simulink model "FSK_mod_demod"  (R2021a)
settings: Solver=VariableStepAuto  StartTime=0.0  StopTime=10  RelTol=1e-3
libraries: fl_lib x93, nesl_utility x28, ee_lib x20
settings Model: Creator=Bharat Gunhalkar  LastModifiedBy=Bharat Gunhalkar

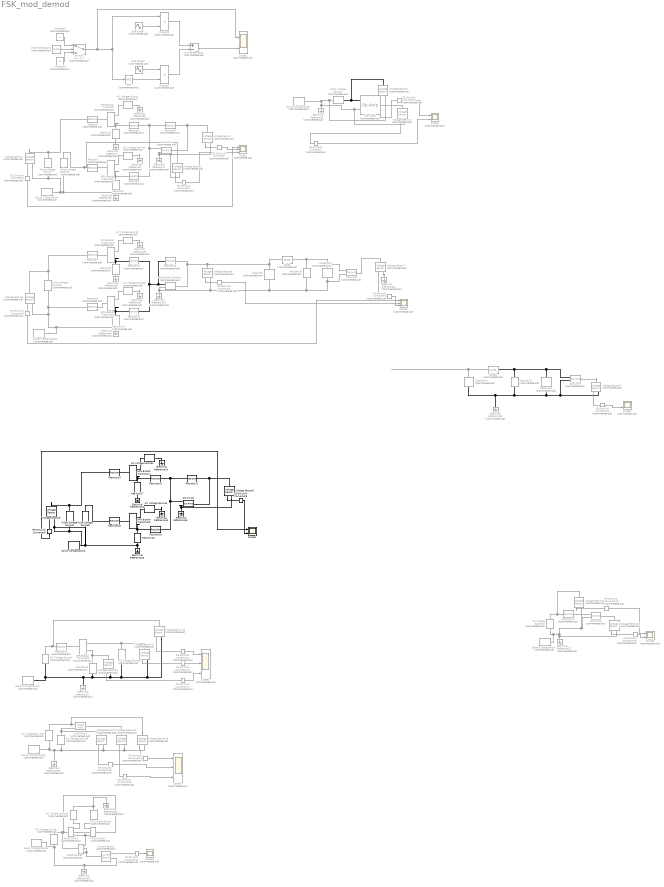
== system FSK_mod_demod ==
  AC Current Source : fl_lib/Electrical/Electrical Sources/AC Current Source  Commented=on  amp=5 A  shift=0 deg  frequency=60 Hz  omega=0 rad/s
      settings: SourceProductBaseCode=SS  InternalSimscapePortConfiguration="{\"Bottom\":[],\"Left\":[{\"id\":\"p\",\"label\":\"\",\"type\":\"foundation.electrical.electrical\"}],\"Right\":[{\"id\":\"n\",\"label\":\"\",\"type\":\"foundation.electrical.electrical\"}],\"Top\":[]}"
  AC Current Source1 : fl_lib/Electrical/Electrical Sources/AC Current Source  Commented=on  amp=2 A  shift=0 deg  frequency=60 Hz  omega=0 rad/s
      settings: SourceProductBaseCode=SS  InternalSimscapePortConfiguration="{\"Bottom\":[],\"Left\":[{\"id\":\"p\",\"label\":\"\",\"type\":\"foundation.electrical.electrical\"}],\"Right\":[{\"id\":\"n\",\"label\":\"\",\"type\":\"foundation.electrical.electrical\"}],\"Top\":[]}"
  AC Voltage Source : fl_lib/Electrical/Electrical Sources/AC Voltage Source  Commented=on  amp=.7 V  shift=90 deg  frequency=100 Hz  omega=0 rad/s
  AC Voltage Source1 : fl_lib/Electrical/Electrical Sources/AC Voltage Source  Commented=on  amp=.7 V  shift=90 deg  frequency=1000 Hz  omega=0 rad/s
  AC Voltage Source10 : fl_lib/Electrical/Electrical Sources/AC Voltage Source  Commented=on  amp=1 V  shift=0 deg  frequency=1 Hz  omega=0 rad/s
  AC Voltage Source2 : fl_lib/Electrical/Electrical Sources/AC Voltage Source  Commented=on  amp=.7 V  shift=90 deg  frequency=200 Hz  omega=0 rad/s
  AC Voltage Source3 : fl_lib/Electrical/Electrical Sources/AC Voltage Source  Commented=on  amp=.7 V  shift=90 deg  frequency=2000 Hz  omega=0 rad/s
  AC Voltage Source4 : fl_lib/Electrical/Electrical Sources/AC Voltage Source  amp=.4 V  shift=90 deg  frequency=10 Hz  omega=0 rad/s
  AC Voltage Source5 : fl_lib/Electrical/Electrical Sources/AC Voltage Source  amp=.4 V  shift=90 deg  frequency=1000 Hz  omega=0 rad/s
  AC Voltage Source6 : fl_lib/Electrical/Electrical Sources/AC Voltage Source  Commented=on  amp=4 V  shift=0 deg  frequency=.5 Hz  omega=0 rad/s
  AC Voltage Source7 : fl_lib/Electrical/Electrical Sources/AC Voltage Source  Commented=on  amp=2 V  shift=0 deg  frequency=.5 Hz  omega=0 rad/s
  AC Voltage Source8 : fl_lib/Electrical/Electrical Sources/AC Voltage Source  Commented=on  amp=2 V  shift=0 deg  frequency=.5 Hz  omega=0 rad/s
  AC Voltage Source9 : fl_lib/Electrical/Electrical Sources/AC Voltage Source  Commented=on  amp=4 V  shift=0 deg  frequency=.5 Hz  omega=0 rad/s
  CMOS AND : ee_lib/Integrated Circuits/Logic/CMOS AND  Commented=on  V_IL=2 V  V_IH=3 V  C_IN=5 pF  output_type=1  V_OL=0 V  V_OH=5 V  V_CC=5 V  V_meas=5 V  R_OUT=25 Ohm  R_OH=[25, 250] Ohm  I_OH=63 mA  R_OL=[30, 800] Ohm  I_OL=-45 mA  Delay=25 ns  Ron=5 Ohm  Vf=0.6 V  output_state=1
      settings: SourceProductBaseCode=PS  InternalSimscapePortConfiguration="{\"Bottom\":[],\"Left\":[{\"id\":\"A\",\"label\":\"\",\"type\":\"foundation.electrical.electrical\"},{\"id\":\"B\",\"label\":\"\",\"type\":\"foundation.electrical.electrical\"}],\"Right\":[{\"id\":\"J\",\"label\":\"\",\"type\":\"foundation.electrical.electrical\"}],\"Top\":[]}"
  Capacitor : fl_lib/Electrical/Electrical Elements/Capacitor  Commented=on  c=0.1e-6 F  r=1e-6 Ohm  g=0 1/Ohm  i_specify=off  i_priority=None  i=0 A  i_nominal_specify=off  i_nominal_unit=A  i_nominal_value=1  v_specify=off  v_priority=None  v=0 V  v_nominal_specify=off  v_nominal_unit=V  v_nominal_value=1  vc_specify=off  vc_priority=High  vc=0 V  vc_nominal_specify=off  vc_nominal_unit=V  vc_nominal_value=1
  Capacitor1 : fl_lib/Electrical/Electrical Elements/Capacitor  Commented=on  c=0.01e-6 F  r=1e-6 Ohm  g=0 1/Ohm  i_specify=off  i_priority=None  i=0 A  i_nominal_specify=off  i_nominal_unit=A  i_nominal_value=1  v_specify=off  v_priority=None  v=0 V  v_nominal_specify=off  v_nominal_unit=V  v_nominal_value=1  vc_specify=off  vc_priority=High  vc=0 V  vc_nominal_specify=off  vc_nominal_unit=V  vc_nominal_value=1
  Capacitor4 : fl_lib/Electrical/Electrical Elements/Capacitor  Commented=on  c=0.1 uF  r=1e-6 Ohm  g=0 1/Ohm  i_specify=off  i_priority=None  i=0 A  i_nominal_specify=off  i_nominal_unit=A  i_nominal_value=1  v_specify=off  v_priority=None  v=0 V  v_nominal_specify=off  v_nominal_unit=V  v_nominal_value=1  vc_specify=off  vc_priority=High  vc=0 V  vc_nominal_specify=off  vc_nominal_unit=V  vc_nominal_value=1
  Capacitor5 : fl_lib/Electrical/Electrical Elements/Capacitor  Commented=on  c=0.01 uF  r=1e-6 Ohm  g=0 1/Ohm  i_specify=off  i_priority=None  i=0 A  i_nominal_specify=off  i_nominal_unit=A  i_nominal_value=1  v_specify=off  v_priority=None  v=0 V  v_nominal_specify=off  v_nominal_unit=V  v_nominal_value=1  vc_specify=off  vc_priority=High  vc=0 V  vc_nominal_specify=off  vc_nominal_unit=V  vc_nominal_value=1
  Constant2 : Constant  Commented=on
  Constant3 : Constant  Commented=on  Value=0
  Current Sensor : fl_lib/Electrical/Electrical Sensors/Current Sensor  Commented=on
  DC Voltage Source : fl_lib/Electrical/Electrical Sources/DC Voltage Source  Commented=on  v0=0.5 V
  Diode : ee_lib/Semiconductors & Converters/Diode  Commented=on  ModelType=ee.enum.diode.modelType.pwl  IfMat=[.07, .12, .19, 1.75, 4.24, 7.32, 11.2; .16, .3, .72, 2.14, 5.02, 8.35, 13.12] A  TjVec=[25, 125] degC  VfVec=[.5, .7, .9, 1.3, 1.7, 2.1, 2.5] V  Vf=0.6 V  Ron=0.3 Ohm  Goff=1e-8 S  prmExp=ee.enum.diode.expParam.useTwo  I12=[.0137, .545] A  V12=[.6, .7] V  IS=1e-12 A  ec=1  I1=0.0137 A  V1=0.6 V  RS=0 Ohm  Tmeas=25 degC  N_series=1  N_parallel=1  Rz=0.3 Ohm  BV=inf V  C_param=ee.enum.diode.capParam.fixed  CJ=5 pF  CJ0=5 pF  VJ=1 V  Mgrad=0.5  Vvec=[.1, 10, 100] V  Cvec=[3.5, 1, .4] pF  FC=0.5  Q_param=ee.enum.diode.recoveryParam.off  iRM=-7.15 A  iF=4 A  didt=-750 A/us  trr_factor=3  trr=115 ns  Qrr=150 nA*s  TT=50 ns  tau=100 ns  T_param=ee.enum.diode.temperatureParam.off  IS_T2=1.25e-7 A  I1_T2=0.245 A  V1_T2=0.5 V  Tmeas2=125 degC  EG_param=ee.enum.diode.egapParam.material_si  EG=1.11 eV  XTI_param=ee.enum.diode.xtiParam.pn  XTI=3  dBVdT=0 V/K  enable_faults=simscape.enum.onoff.off  fault_action=simscape.enum.assert.action.none  fault_types=ee.enum.diode.faults.open  tau_fault=1e-3 s  IfMat_faulted=[.07, .12, .19, 1.75, 4.24, 7.32, 11.2; .16, .3, .72, 2.14, 4.02, 6.35, 9.12] A  VfVec_faulted=[.5, .7, .9, 1.3, 1.7, 2.1, 2.5] V  Ropen_faulted=1000 Ohm  Gshort_faulted=1000 1/Ohm  Vf_faulted=0.6 V  Ron_faulted=0.3 Ohm  Goff_faulted=1e-8 S  I12_faulted=[.0137, .545] A  V12_faulted=[.6, .7] V  IS_faulted=1e-12 A  ec_faulted=1  I1_faulted=0.0137 A  V1_faulted=0.6 V  RS_faulted=0 Ohm  Rz_faulted=0.3 Ohm  BV_faulted=inf V  Cscale_faulted=100  enable_temporal_fault=simscape.enum.onoff.off  t_fault=inf s  enable_behavioral_fault=simscape.enum.onoff.off  max_permissible_voltage=inf V  n_fail_on_voltage=1  max_permissible_current=inf A  t_fail_on_current=1 s  max_permissible_dVdt=inf V/s  Tdevice=25 degC  i_specify=off  i_priority=None  i=0 A  i_nominal_specify=off  i_nominal_unit=A  i_nominal_value=1  v_specify=off  v_priority=None  v=0 V  v_nominal_specify=off  v_nominal_unit=V  v_nominal_value=1  i_diode_specify=off  i_diode_priority=None  i_diode=0 A  i_diode_nominal_specify=off  i_diode_nominal_unit=A  i_diode_nominal_value=1  v_diode_specify=off  v_diode_priority=None  v_diode=0 V  v_diode_nominal_specify=off  v_diode_nominal_unit=V  v_diode_nominal_value=1  i_capacitor_specify=off  i_capacitor_priority=None  i_capacitor=0 A  i_capacitor_nominal_specify=off  i_capacitor_nominal_unit=A  i_capacitor_nominal_value=1  v_capacitor_specify=off  v_capacitor_priority=None  v_capacitor=0 V  v_capacitor_nominal_specify=off  v_capacitor_nominal_unit=V  v_capacitor_nominal_value=1  power_dissipated_specify=off  power_dissipated_priority=None  power_dissipated=0 W  power_dissipated_nominal_specify=off  power_dissipated_nominal_unit=W  power_dissipated_nominal_value=1  max_permissible_temperature=inf K  t_fail_on_temperature=1 s  thermal_network_parameterization=ee.enum.thermalNetworkTopology.junctionCase  Rth=[0, 10] K/W  Rth_Foster=[4, 6] K/W  thermal_mass_parameterization=ee.enum.thermalNetwork.timeconstant  thermal_mass=[0, 1] J/K  thermal_mass_Foster=[1.5, 3] J/K  thermal_time_constant=[0, 10] s  thermal_time_constant_Foster=[6, 18] s  thermal_mass_initial_temperatures=[25, 25] degC
  Diode2 : ee_lib/Semiconductors & Converters/Diode  Commented=on  ModelType=ee.enum.diode.modelType.pwl  IfMat=[.07, .12, .19, 1.75, 4.24, 7.32, 11.2; .16, .3, .72, 2.14, 4.02, 6.35, 9.12] A  TjVec=[25, 125] degC  VfVec=[.5, .7, .9, 1.3, 1.7, 2.1, 2.5] V  Vf=0.6 V  Ron=0.3 Ohm  Goff=1e-8 S  prmExp=ee.enum.diode.expParam.useTwo  I12=[.0137, .545] A  V12=[.6, .7] V  IS=1e-12 A  ec=1  I1=0.0137 A  V1=0.6 V  RS=0 Ohm  Tmeas=25 degC  N_series=1  N_parallel=1  Rz=0.3 Ohm  BV=inf V  C_param=ee.enum.diode.capParam.fixed  CJ=5 pF  CJ0=5 pF  VJ=1 V  Mgrad=0.5  Vvec=[.1, 10, 100] V  Cvec=[3.5, 1, .4] pF  FC=0.5  Q_param=ee.enum.diode.recoveryParam.off  iRM=-7.15 A  iF=4 A  didt=-750 A/us  trr_factor=3  trr=115 ns  Qrr=150 s*nA  TT=50 ns  tau=100 ns  T_param=ee.enum.diode.temperatureParam.off  IS_T2=1.25e-7 A  I1_T2=0.245 A  V1_T2=0.5 V  Tmeas2=125 degC  EG_param=ee.enum.diode.egapParam.material_si  EG=1.11 eV  XTI_param=ee.enum.diode.xtiParam.pn  XTI=3  dBVdT=0 V/K  enable_faults=ee.enum.faults.faultEnable.no  fault_action=ee.enum.faults.faultAction.none  fault_types=ee.enum.diode.faults.open  tau_fault=1e-3 s  IfMat_faulted=[.07, .12, .19, 1.75, 4.24, 7.32, 11.2; .16, .3, .72, 2.14, 4.02, 6.35, 9.12] A  VfVec_faulted=[.5, .7, .9, 1.3, 1.7, 2.1, 2.5] V  Ropen_faulted=1000 Ohm  Gshort_faulted=1000 1/Ohm  Vf_faulted=0.6 V  Ron_faulted=0.3 Ohm  Goff_faulted=1e-8 S  I12_faulted=[.0137, .545] A  V12_faulted=[.6, .7] V  IS_faulted=1e-12 A  ec_faulted=1  I1_faulted=0.0137 A  V1_faulted=0.6 V  RS_faulted=0 Ohm  Rz_faulted=0.3 Ohm  BV_faulted=inf V  Cscale_faulted=100  enable_temporal_fault=ee.enum.faults.faultEnable.no  t_fault=inf s  enable_behavioral_fault=ee.enum.faults.faultEnable.no  max_permissible_voltage=inf V  n_fail_on_voltage=1  max_permissible_current=inf A  t_fail_on_current=1 s  max_permissible_dVdt=inf V/s  Tdevice=25 degC  i_specify=off  i_priority=None  i=0 A  i_nominal_specify=off  i_nominal_unit=A  i_nominal_value=1  v_specify=off  v_priority=None  v=0 V  v_nominal_specify=off  v_nominal_unit=V  v_nominal_value=1  i_diode_specify=off  i_diode_priority=None  i_diode=0 A  i_diode_nominal_specify=off  i_diode_nominal_unit=A  i_diode_nominal_value=1  v_diode_specify=off  v_diode_priority=None  v_diode=0 V  v_diode_nominal_specify=off  v_diode_nominal_unit=V  v_diode_nominal_value=1  i_capacitor_specify=off  i_capacitor_priority=None  i_capacitor=0 A  i_capacitor_nominal_specify=off  i_capacitor_nominal_unit=A  i_capacitor_nominal_value=1  v_capacitor_specify=off  v_capacitor_priority=None  v_capacitor=0 V  v_capacitor_nominal_specify=off  v_capacitor_nominal_unit=V  v_capacitor_nominal_value=1  power_dissipated_specify=off  power_dissipated_priority=None  power_dissipated=0 W  power_dissipated_nominal_specify=off  power_dissipated_nominal_unit=W  power_dissipated_nominal_value=1  max_permissible_temperature=inf K  t_fail_on_temperature=1 s  thermal_network_parameterization=ee.enum.thermalNetworkTopology.cauer  Rth=[0, 10] K/W  Rth_Foster=[4, 6] K/W  thermal_mass_parameterization=ee.enum.thermalNetwork.timeconstant  thermal_mass=[0, 1] J/K  thermal_mass_Foster=[1.5, 3] J/K  thermal_time_constant=[0, 10] s  thermal_time_constant_Foster=[6, 18] s  thermal_mass_initial_temperatures=[25, 25] degC
  Electrical Reference{,1..11,17..22} (18 alike) : fl_lib/Electrical/Electrical Elements/Electrical Reference  Commented=on
  Electrical Reference{12..16} (5 alike) : fl_lib/Electrical/Electrical Elements/Electrical Reference
  Finite-Gain Op-Amp : ee_lib/Integrated Circuits/Finite-Gain Op-Amp  Commented=on  A=1000  Rin=1e30 Ohm  Rout=1000 Ohm  Vmin=-15 V  Vmax=15 V  noise_mode=0  v_noise=30e-9 V/Hz^(1/2)  noise_prm=1  i_noise=0.5e-12 A/Hz^(1/2)  ip_noise=0.5e-12 A/Hz^(1/2)  in_noise=0.5e-12 A/Hz^(1/2)  sample_time=1e-3 s  repeatability=1  auto_seed_v=1792148415  auto_seed_ip=213264155  auto_seed_in=3877136169  user_seed_v=0  user_seed_ip=0  user_seed_in=0
      settings: SourceProductBaseCode=PS  InternalSimscapePortConfiguration="{\"Bottom\":[],\"Left\":[{\"id\":\"p\",\"label\":\"+\",\"type\":\"foundation.electrical.electrical\"},{\"id\":\"n\",\"label\":\"-\",\"type\":\"foundation.electrical.electrical\"}],\"Right\":[{\"id\":\"out\",\"label\":\"\",\"type\":\"foundation.electrical.electrical\"}],\"Top\":[]}"
  NOT : Logic  Commented=on  Operator=NOT  IconShape=distinctive  AllPortsSameDT=off  OutDataTypeStr=boolean
  NPN Bipolar Transistor{,1..3} (4 alike) : ee_lib/Semiconductors & Converters/NPN Bipolar Transistor  Commented=on  parameterization=1  prmDatasheet=1  prmEquCoeff=1  BF=100  IS=1e-14 A  VAF=200 V  hfe=100  hoe=50e-6 1/Ohm  Ic_h=1 mA  Vce_h=5 V  V1=0.55 V  I1=0.5 mA  BR=1  Tmeas=25 degC  RC=0.01 Ohm  RE=1e-4 Ohm  RB=1 Ohm  C_BC=5 pF  C_BE=5 pF  TF=0 us  TR=0 us  hfe_T2=125  XTB=0  V1_T2=0.45 V  I1_T2=0.5 mA  Tmeas2=125 degC  EG=1.11 eV  XTI=3  ec=1  TdeviceDatasheet=25 degC  TdeviceEquCoeff=25 degC  thermal_network_parameterization=ee.enum.thermalNetworkTopology.junctionCase  Rth=[0, 10] K/W  Rth_Foster=[4, 6] K/W  thermal_mass_parameterization=ee.enum.thermalNetwork.timeconstant  thermal_mass=[0, 1] J/K  thermal_mass_Foster=[1.5, 3] J/K  thermal_time_constant=[0, 10] s  thermal_time_constant_Foster=[6, 18] s  thermal_mass_initial_temperatures=[25, 25] degC
  NPN Bipolar Transistor4 : ee_lib/Semiconductors & Converters/NPN Bipolar Transistor  parameterization=1  prmDatasheet=1  prmEquCoeff=1  BF=100  IS=1e-14 A  VAF=200 V  hfe=100  hoe=50e-6 1/Ohm  Ic_h=1 mA  Vce_h=5 V  V1=0.55 V  I1=0.5 mA  BR=1  Tmeas=25 degC  RC=0.01 Ohm  RE=1e-4 Ohm  RB=1 Ohm  C_BC=5 pF  C_BE=5 pF  TF=0 us  TR=0 us  hfe_T2=125  XTB=0  V1_T2=0.45 V  I1_T2=0.5 mA  Tmeas2=125 degC  EG=1.11 eV  XTI=3  ec=1  TdeviceDatasheet=25 degC  TdeviceEquCoeff=25 degC  thermal_network_parameterization=ee.enum.thermalNetworkTopology.junctionCase  Rth=[0, 10] K/W  Rth_Foster=[4, 6] K/W  thermal_mass_parameterization=ee.enum.thermalNetwork.timeconstant  thermal_mass=[0, 1] J/K  thermal_mass_Foster=[1.5, 3] J/K  thermal_time_constant=[0, 10] s  thermal_time_constant_Foster=[6, 18] s  thermal_mass_initial_temperatures=[25, 25] degC
  NPN Bipolar Transistor5 : ee_lib/Semiconductors & Converters/NPN Bipolar Transistor  parameterization=1  prmDatasheet=1  prmEquCoeff=1  BF=100  IS=1e-14 A  VAF=200 V  hfe=100  hoe=50e-6 1/Ohm  Ic_h=1 mA  Vce_h=5 V  V1=0.55 V  I1=0.5 mA  BR=1  Tmeas=25 degC  RC=0.01 Ohm  RE=1e-4 Ohm  RB=1 Ohm  C_BC=5 pF  C_BE=5 pF  TF=0 us  TR=0 us  hfe_T2=125  XTB=0  V1_T2=0.45 V  I1_T2=0.5 mA  Tmeas2=125 degC  EG=1.11 eV  XTI=3  ec=1  TdeviceDatasheet=25 degC  TdeviceEquCoeff=25 degC  thermal_network_parameterization=ee.enum.thermalNetworkTopology.junctionCase  Rth=[0, 10] K/W  Rth_Foster=[4, 6] K/W  thermal_mass_parameterization=ee.enum.thermalNetwork.timeconstant  thermal_mass=[0, 1] J/K  thermal_mass_Foster=[1.5, 3] J/K  thermal_time_constant=[0, 10] s  thermal_time_constant_Foster=[6, 18] s  thermal_mass_initial_temperatures=[25, 25] degC
  NPN Bipolar Transistor6 : ee_lib/Semiconductors & Converters/NPN Bipolar Transistor  Commented=on  parameterization=1  prmDatasheet=1  prmEquCoeff=1  BF=100  IS=1e-14 A  VAF=200 V  hfe=100  hoe=50e-6 1/Ohm  Ic_h=1 mA  Vce_h=5 V  V1=0.55 V  I1=0.5 mA  BR=1  Tmeas=25 degC  RC=0.01 Ohm  RE=1e-4 Ohm  RB=1 Ohm  C_BC=5 pF  C_BE=5 pF  TF=0 us  TR=0 us  hfe_T2=125  XTB=0  V1_T2=0.45 V  I1_T2=0.5 mA  Tmeas2=125 degC  EG=1.11 eV  XTI=3  ec=1  TdeviceDatasheet=25 degC  TdeviceEquCoeff=25 degC  thermal_network_parameterization=ee.enum.thermalNetworkTopology.cauer  Rth=[0, 10] K/W  Rth_Foster=[4, 6] K/W  thermal_mass_parameterization=ee.enum.thermalNetwork.timeconstant  thermal_mass=[0, 1] J/K  thermal_mass_Foster=[1.5, 3] J/K  thermal_time_constant=[0, 10] s  thermal_time_constant_Foster=[6, 18] s  thermal_mass_initial_temperatures=[25, 25] degC
  Op-Amp{,1,4..5} (4 alike) : fl_lib/Electrical/Electrical Elements/Op-Amp  Commented=on  outI_specify=off  outI_priority=None  outI=0 A  outI_nominal_specify=off  outI_nominal_unit=A  outI_nominal_value=1
  Op-Amp2 : fl_lib/Electrical/Electrical Elements/Op-Amp  Commented=on  outI_specify=on  outI_priority=None  outI=0 A  outI_nominal_specify=off  outI_nominal_unit=A  outI_nominal_value=1
  Op-Amp3 : fl_lib/Electrical/Electrical Elements/Op-Amp  outI_specify=off  outI_priority=None  outI=0 A  outI_nominal_specify=off  outI_nominal_unit=A  outI_nominal_value=1
  PS-Simulink Converter{,1..7,11..20} (18 alike) : nesl_utility/PS-Simulink Converter  Commented=on  PhysicalDomain=network_engine_domain  SubClassName=ps_output  LeftPortType=input  RightPortType=output  PseudoPeriodic=off  Frequencies=[]  Unit=inherit  AffineConversion=off
      settings: SourceProductBaseCode=PW,SS
  PS-Simulink Converter8 : nesl_utility/PS-Simulink Converter  PhysicalDomain=network_engine_domain  SubClassName=ps_output  LeftPortType=input  RightPortType=output  PseudoPeriodic=off  Frequencies=[]  Unit=inherit  AffineConversion=off
      settings: SourceProductBaseCode=PW,SS
  PS-Simulink Converter9 : nesl_utility/PS-Simulink Converter  PhysicalDomain=network_engine_domain  SubClassName=ps_output  LeftPortType=input  RightPortType=output  PseudoPeriodic=off  Frequencies=[]  Unit=inherit  AffineConversion=off
      settings: SourceProductBaseCode=PW,SS
  Product1 : Product  Commented=on
  Product2 : Product  Commented=on
  Pulse Generator1 : DiscretePulseGenerator  Commented=on  PulseType=Time based  PulseWidth=50
  Pulse Voltage Source : ee_lib/Additional Components/SPICE Sources/Pulse Voltage Source  Commented=on  V1=0 V  V2=1 V  TD=0 s  TR=1e-9 s  TF=1e-9 s  PW=.5 s  PER=1 s
      settings: SourceProductBaseCode=PS  InternalSimscapePortConfiguration="{\"Bottom\":[],\"Left\":[{\"id\":\"p\",\"label\":\"\",\"type\":\"foundation.electrical.electrical\"}],\"Right\":[{\"id\":\"n\",\"label\":\"\",\"type\":\"foundation.electrical.electrical\"}],\"Top\":[]}"
  Pulse Voltage Source1 : ee_lib/Additional Components/SPICE Sources/Pulse Voltage Source  Commented=on  V1=0 V  V2=0 V  TD=0 s  TR=1e-9 s  TF=1e-9 s  PW=Inf s  PER=Inf s
      settings: SourceProductBaseCode=PS  InternalSimscapePortConfiguration="{\"Bottom\":[],\"Left\":[{\"id\":\"p\",\"label\":\"\",\"type\":\"foundation.electrical.electrical\"}],\"Right\":[{\"id\":\"n\",\"label\":\"\",\"type\":\"foundation.electrical.electrical\"}],\"Top\":[]}"
  Pulse Voltage Source2 : ee_lib/Additional Components/SPICE Sources/Pulse Voltage Source  Commented=on  V1=1 V  V2=0 V  TD=0 s  TR=1e-9 s  TF=1e-9 s  PW=.5 s  PER=1 s
      settings: SourceProductBaseCode=PS  InternalSimscapePortConfiguration="{\"Bottom\":[],\"Left\":[{\"id\":\"p\",\"label\":\"\",\"type\":\"foundation.electrical.electrical\"}],\"Right\":[{\"id\":\"n\",\"label\":\"\",\"type\":\"foundation.electrical.electrical\"}],\"Top\":[]}"
  Pulse Voltage Source3 : ee_lib/Additional Components/SPICE Sources/Pulse Voltage Source  Commented=on  V1=0 V  V2=1 V  TD=0 s  TR=1e-9 s  TF=1e-9 s  PW=.5 s  PER=1 s
      settings: SourceProductBaseCode=PS  InternalSimscapePortConfiguration="{\"Bottom\":[],\"Left\":[{\"id\":\"p\",\"label\":\"\",\"type\":\"foundation.electrical.electrical\"}],\"Right\":[{\"id\":\"n\",\"label\":\"\",\"type\":\"foundation.electrical.electrical\"}],\"Top\":[]}"
  Pulse Voltage Source4 : ee_lib/Additional Components/SPICE Sources/Pulse Voltage Source  V1=0 V  V2=1 V  TD=0 s  TR=1e-9 s  TF=1e-9 s  PW=.5 s  PER=1 s
      settings: SourceProductBaseCode=PS  InternalSimscapePortConfiguration="{\"Bottom\":[],\"Left\":[{\"id\":\"p\",\"label\":\"\",\"type\":\"foundation.electrical.electrical\"}],\"Right\":[{\"id\":\"n\",\"label\":\"\",\"type\":\"foundation.electrical.electrical\"}],\"Top\":[]}"
  Pulse Voltage Source5 : ee_lib/Additional Components/SPICE Sources/Pulse Voltage Source  V1=1 V  V2=0 V  TD=0 s  TR=1e-9 s  TF=1e-9 s  PW=.5 s  PER=1 s
      settings: SourceProductBaseCode=PS  InternalSimscapePortConfiguration="{\"Bottom\":[],\"Left\":[{\"id\":\"p\",\"label\":\"\",\"type\":\"foundation.electrical.electrical\"}],\"Right\":[{\"id\":\"n\",\"label\":\"\",\"type\":\"foundation.electrical.electrical\"}],\"Top\":[]}"
  Resistor{,1,7..8} (4 alike) : fl_lib/Electrical/Electrical Elements/Resistor  Commented=on  R=1 kOhm  i_specify=off  i_priority=None  i=0 A  i_nominal_specify=off  i_nominal_unit=A  i_nominal_value=1  v_specify=off  v_priority=None  v=0 V  v_nominal_specify=off  v_nominal_unit=V  v_nominal_value=1
  Resistor{2..3,9..10,24} (5 alike) : fl_lib/Electrical/Electrical Elements/Resistor  Commented=on  R=2200 Ohm  i_specify=off  i_priority=None  i=0 A  i_nominal_specify=off  i_nominal_unit=A  i_nominal_value=1  v_specify=off  v_priority=None  v=0 V  v_nominal_specify=off  v_nominal_unit=V  v_nominal_value=1
  Resistor{4..6,11..13} (6 alike) : fl_lib/Electrical/Electrical Elements/Resistor  Commented=on  R=10000 Ohm  i_specify=off  i_priority=None  i=0 A  i_nominal_specify=off  i_nominal_unit=A  i_nominal_value=1  v_specify=off  v_priority=None  v=0 V  v_nominal_specify=off  v_nominal_unit=V  v_nominal_value=1
  Resistor14 : fl_lib/Electrical/Electrical Elements/Resistor  Commented=on  R=50000 Ohm  i_specify=off  i_priority=None  i=0 A  i_nominal_specify=off  i_nominal_unit=A  i_nominal_value=1  v_specify=off  v_priority=None  v=0 V  v_nominal_specify=off  v_nominal_unit=V  v_nominal_value=1
  Resistor15 : fl_lib/Electrical/Electrical Elements/Resistor  R=1 kOhm  i_specify=off  i_priority=None  i=0 A  i_nominal_specify=off  i_nominal_unit=A  i_nominal_value=1  v_specify=off  v_priority=None  v=0 V  v_nominal_specify=off  v_nominal_unit=V  v_nominal_value=1
  Resistor16 : fl_lib/Electrical/Electrical Elements/Resistor  R=1 kOhm  i_specify=off  i_priority=None  i=0 A  i_nominal_specify=off  i_nominal_unit=A  i_nominal_value=1  v_specify=off  v_priority=None  v=0 V  v_nominal_specify=off  v_nominal_unit=V  v_nominal_value=1
  Resistor17 : fl_lib/Electrical/Electrical Elements/Resistor  R=2200 Ohm  i_specify=off  i_priority=None  i=0 A  i_nominal_specify=off  i_nominal_unit=A  i_nominal_value=1  v_specify=off  v_priority=None  v=0 V  v_nominal_specify=off  v_nominal_unit=V  v_nominal_value=1
  Resistor18 : fl_lib/Electrical/Electrical Elements/Resistor  R=2200 Ohm  i_specify=off  i_priority=None  i=0 A  i_nominal_specify=off  i_nominal_unit=A  i_nominal_value=1  v_specify=off  v_priority=None  v=0 V  v_nominal_specify=off  v_nominal_unit=V  v_nominal_value=1
  Resistor19 : fl_lib/Electrical/Electrical Elements/Resistor  R=10000 Ohm  i_specify=off  i_priority=None  i=0 A  i_nominal_specify=off  i_nominal_unit=A  i_nominal_value=1  v_specify=off  v_priority=None  v=0 V  v_nominal_specify=off  v_nominal_unit=V  v_nominal_value=1
  Resistor20 : fl_lib/Electrical/Electrical Elements/Resistor  R=10000 Ohm  i_specify=off  i_priority=None  i=0 A  i_nominal_specify=off  i_nominal_unit=A  i_nominal_value=1  v_specify=off  v_priority=None  v=0 V  v_nominal_specify=off  v_nominal_unit=V  v_nominal_value=1
  Resistor21 : fl_lib/Electrical/Electrical Elements/Resistor  R=10000 Ohm  i_specify=off  i_priority=None  i=0 A  i_nominal_specify=off  i_nominal_unit=A  i_nominal_value=1  v_specify=off  v_priority=None  v=0 V  v_nominal_specify=off  v_nominal_unit=V  v_nominal_value=1
  Resistor22 : fl_lib/Electrical/Electrical Elements/Resistor  Commented=on  R=1 Ohm  i_specify=off  i_priority=None  i=0 A  i_nominal_specify=off  i_nominal_unit=A  i_nominal_value=1  v_specify=off  v_priority=None  v=0 V  v_nominal_specify=off  v_nominal_unit=V  v_nominal_value=1
  Resistor23 : fl_lib/Electrical/Electrical Elements/Resistor  Commented=on  R=50000 Ohm  i_specify=off  i_priority=None  i=0 A  i_nominal_specify=off  i_nominal_unit=A  i_nominal_value=1  v_specify=off  v_priority=None  v=0 V  v_nominal_specify=off  v_nominal_unit=V  v_nominal_value=1
  Resistor25 : fl_lib/Electrical/Electrical Elements/Resistor  Commented=on  R=1000 Ohm  i_specify=off  i_priority=None  i=0 A  i_nominal_specify=off  i_nominal_unit=A  i_nominal_value=1  v_specify=off  v_priority=None  v=0 V  v_nominal_specify=off  v_nominal_unit=V  v_nominal_value=1
  SPICE NMOS : ee_lib/Additional Components/SPICE Semiconductors/SPICE NMOS  Commented=on  AREA=1.0  SCALE=1  LENGTH=1 um  WIDTH=10 um  AD=0 m^2  AS=0 m^2  PD=0 m  PS=0 m  NRD=0  NRS=0  LEVEL=1  VTO=0.4 V  KP=2e-5 A/V^2  GAMMA=0 V^0.50000  PHI=0.6 V  LAMBDA=0 1/V  RD=0 Ohm  RS=0 Ohm  Ci_param=ee.enum.intrinsicCapacitance.none  Cov_param=ee.enum.includeCapacitance.no  CGSO=0 F/m  CGDO=0 F/m  CGBO=0 F/m  C_param=ee.enum.includeCapacitance.no  CBD=0 F  CBS=0 F  IS=1e-14 A  N=1  PB=0.8 V  RSH=0 Ohm  CJ=0 F/m^2  MJ=0.5  CJSW=0 F/m  MJSW=0.5  JS=0 A/m^2  TOX=1e-7 m  LD=0 m  U0=600 cm^2/s/V  FC=0.5  NSUB=NaN 1/cm^3  TPG=1  NSS=NaN 1/cm^2  DELTA=0  VMAX=0 m/s  XJ=0 m  NFS=0 1/cm^2  ETA=0  THETA=0 1/V  KAPPA=0.2  T_param=1  TFIXED=300.15 K  TMEAS=300.15 K  TOFFSET=0 K  UEXP=0  UCRIT=1e4 V/cm  NEFF=1  IC_given=ee.enum.initialCondition.no  ICVDS=0 V  ICVGS=0 V  ICVBS=0 V  MTYPE=1
      settings: SourceProductBaseCode=PS  InternalSimscapePortConfiguration="{\"Bottom\":[],\"Left\":[{\"id\":\"gx\",\"label\":\"\",\"type\":\"foundation.electrical.electrical\"}],\"Right\":[{\"id\":\"dx\",\"label\":\"\",\"type\":\"foundation.electrical.electrical\"},{\"id\":\"bx\",\"label\":\"\",\"type\":\"foundation.electrical.electrical\"},{\"id\":\"sx\",\"label\":\"\",\"type\":\"foundation.electrical.electrical\"}],\"Top\":[]}"
  SPICE NMOS1 : ee_lib/Additional Components/SPICE Semiconductors/SPICE NMOS  Commented=on  AREA=1.0  SCALE=1  LENGTH=1 um  WIDTH=10 um  AD=0 m^2  AS=0 m^2  PD=0 m  PS=0 m  NRD=0  NRS=0  LEVEL=1  VTO=.4 V  KP=2e-5 A/V^2  GAMMA=0 V^0.50000  PHI=0.6 V  LAMBDA=0 1/V  RD=0 Ohm  RS=0 Ohm  Ci_param=ee.enum.intrinsicCapacitance.none  Cov_param=ee.enum.includeCapacitance.no  CGSO=0 F/m  CGDO=0 F/m  CGBO=0 F/m  C_param=ee.enum.includeCapacitance.no  CBD=0 F  CBS=0 F  IS=1e-14 A  N=1  PB=0.8 V  RSH=0 Ohm  CJ=0 F/m^2  MJ=0.5  CJSW=0 F/m  MJSW=0.5  JS=0 A/m^2  TOX=1e-7 m  LD=0 m  U0=600 cm^2/s/V  FC=0.5  NSUB=NaN 1/cm^3  TPG=1  NSS=NaN 1/cm^2  DELTA=0  VMAX=0 m/s  XJ=0 m  NFS=0 1/cm^2  ETA=0  THETA=0 1/V  KAPPA=0.2  T_param=1  TFIXED=300.15 K  TMEAS=300.15 K  TOFFSET=0 K  UEXP=0  UCRIT=1e4 V/cm  NEFF=1  IC_given=ee.enum.initialCondition.no  ICVDS=0 V  ICVGS=0 V  ICVBS=0 V  MTYPE=1
      settings: SourceProductBaseCode=PS  InternalSimscapePortConfiguration="{\"Bottom\":[],\"Left\":[{\"id\":\"gx\",\"label\":\"\",\"type\":\"foundation.electrical.electrical\"}],\"Right\":[{\"id\":\"dx\",\"label\":\"\",\"type\":\"foundation.electrical.electrical\"},{\"id\":\"bx\",\"label\":\"\",\"type\":\"foundation.electrical.electrical\"},{\"id\":\"sx\",\"label\":\"\",\"type\":\"foundation.electrical.electrical\"}],\"Top\":[]}"
  SPICE NMOS2 : ee_lib/Additional Components/SPICE Semiconductors/SPICE NMOS  Commented=on  AREA=1.0  SCALE=1  LENGTH=1 um  WIDTH=10 um  AD=0 m^2  AS=0 m^2  PD=0 m  PS=0 m  NRD=0  NRS=0  LEVEL=1  VTO=.4 V  KP=2e-5 A/V^2  GAMMA=0 V^0.50000  PHI=0.6 V  LAMBDA=0 1/V  RD=0 Ohm  RS=0 Ohm  Ci_param=ee.enum.intrinsicCapacitance.none  Cov_param=ee.enum.includeCapacitance.no  CGSO=0 F/m  CGDO=0 F/m  CGBO=0 F/m  C_param=ee.enum.includeCapacitance.no  CBD=0 F  CBS=0 F  IS=1e-14 A  N=1  PB=0.8 V  RSH=0 Ohm  CJ=0 F/m^2  MJ=0.5  CJSW=0 F/m  MJSW=0.5  JS=0 A/m^2  TOX=1e-7 m  LD=0 m  U0=600 cm^2/s/V  FC=0.5  NSUB=NaN 1/cm^3  TPG=1  NSS=NaN 1/cm^2  DELTA=0  VMAX=0 m/s  XJ=0 m  NFS=0 1/cm^2  ETA=0  THETA=0 1/V  KAPPA=0.2  T_param=1  TFIXED=300.15 K  TMEAS=300.15 K  TOFFSET=0 K  UEXP=0  UCRIT=1e4 V/cm  NEFF=1  IC_given=ee.enum.initialCondition.no  ICVDS=0 V  ICVGS=0 V  ICVBS=0 V  MTYPE=1
      settings: SourceProductBaseCode=PS  InternalSimscapePortConfiguration="{\"Bottom\":[],\"Left\":[{\"id\":\"gx\",\"label\":\"\",\"type\":\"foundation.electrical.electrical\"}],\"Right\":[{\"id\":\"dx\",\"label\":\"\",\"type\":\"foundation.electrical.electrical\"},{\"id\":\"bx\",\"label\":\"\",\"type\":\"foundation.electrical.electrical\"},{\"id\":\"sx\",\"label\":\"\",\"type\":\"foundation.electrical.electrical\"}],\"Top\":[]}"
  Scope{,3,5,7} (4 alike) : Scope  Commented=on  NumInputPorts=3
  Scope{1..2,6,9} (4 alike) : Scope  Commented=on  NumInputPorts=2
  Scope4 : Scope  NumInputPorts=2
  Scope8 : Scope  Commented=on
  Sine Wave1 : Sin  Commented=on  Amplitude=14.142  Frequency=2*pi*100  Phase=90  SampleTime=0
  Sine Wave2 : Sin  Commented=on  Amplitude=14.142  Frequency=2*pi*1000  Phase=90  SampleTime=0
  Solver Configuration{,1..2,4..7} (7 alike) : nesl_utility/Solver Configuration  Commented=on  PhysicalDomain=network_engine_domain  SubClassName=solver  LeftPortType=input  RightPortType=generic  Tones=[]  Harmonics=[]  SimulateNoise=off  Profile=off  UseLocalSampling=off  EnableSwitchedLinearOptims=on  FrequencyDomain=off  UseCCode=off  RelTol=0.001  AbsTol=1e-06  MinStep=1e-09  ToWorkspace=off  RevertToSquareIcSolve=off  NumHomotopyIterations=100  PhasorMode=off  PhasorModeNumHarmonics=1  DoDC=off  ResidualTolerance=1e-09  UseLocalSolver=off  LocalSolverChoice=NE_BACKWARD_EULER_ADVANCER  LocalSolverSampleTime=0.001  DoFixedCost=off  MaxNonlinIter=3  MaxModeIter=2  ComputeImpulses=off  ImpulseIterations=2  LinearAlgebra=auto  EquationFormulation=NE_TIME_EF  DelaysMemoryBudget=1024  AutomaticFiltering=on  FilteringTimeConstant=0.001  PartitionStorageMethod=AS_NEEDED  PartitionMemoryBudget=1024  PartitionMethod=ROBUST
      settings: SourceProductBaseCode=PW,SS
  Solver Configuration3 : nesl_utility/Solver Configuration  PhysicalDomain=network_engine_domain  SubClassName=solver  LeftPortType=input  RightPortType=generic  Tones=[]  Harmonics=[]  SimulateNoise=off  Profile=off  UseLocalSampling=off  EnableSwitchedLinearOptims=on  FrequencyDomain=off  UseCCode=off  RelTol=0.001  AbsTol=1e-06  MinStep=1e-09  ToWorkspace=off  RevertToSquareIcSolve=off  NumHomotopyIterations=100  PhasorMode=off  PhasorModeNumHarmonics=1  DoDC=off  ResidualTolerance=1e-09  UseLocalSolver=off  LocalSolverChoice=NE_BACKWARD_EULER_ADVANCER  LocalSolverSampleTime=0.001  DoFixedCost=off  MaxNonlinIter=3  MaxModeIter=2  ComputeImpulses=off  ImpulseIterations=2  LinearAlgebra=auto  EquationFormulation=NE_TIME_EF  DelaysMemoryBudget=1024  AutomaticFiltering=on  FilteringTimeConstant=0.001  PartitionStorageMethod=AS_NEEDED  PartitionMemoryBudget=1024  PartitionMethod=ROBUST
      settings: SourceProductBaseCode=PW,SS
  Sum of Elements : Sum  Commented=on  Inputs=+-
  Switch1 : Switch  Commented=on  Threshold=1
  Voltage Sensor{,1..7,11..19} (17 alike) : fl_lib/Electrical/Electrical Sensors/Voltage Sensor  Commented=on
  Voltage Sensor8 : fl_lib/Electrical/Electrical Sensors/Voltage Sensor
  Voltage Sensor9 : fl_lib/Electrical/Electrical Sensors/Voltage Sensor
  wires:
  Pulse Generator1/1 -> Switch1/2
  Constant2/1 -> Switch1/1
  Constant3/1 -> Switch1/3
  Switch1/1 -> Scope2/1, NOT/1, Product1/1
  Sine Wave1/1 -> Product1/2
  Sine Wave2/1 -> Product2/1
  Product1/1 -> Sum of Elements/1
  Product2/1 -> Sum of Elements/2
  Sum of Elements/1 -> Scope2/2
  NOT/1 -> Product2/2
  PS-Simulink Converter/1 -> Scope/2
  PS-Simulink Converter1/1 -> Scope/1
  PS-Simulink Converter2/1 -> Scope1/2
  PS-Simulink Converter3/1 -> Scope1/1
  PS-Simulink Converter4/1 -> Scope/3
  PS-Simulink Converter6/1 -> Scope3/1
  PS-Simulink Converter5/1 -> Scope3/2
  PS-Simulink Converter7/1 -> Scope3/3
  PS-Simulink Converter8/1 -> Scope4/2
  PS-Simulink Converter9/1 -> Scope4/1
  ? -> Scope6/1
  PS-Simulink Converter12/1 -> Scope6/2
  PS-Simulink Converter11/1 -> Scope5/1
  PS-Simulink Converter14/1 -> Scope5/3
  PS-Simulink Converter13/1 -> Scope5/2
  PS-Simulink Converter17/1 -> Scope7/1
  PS-Simulink Converter15/1 -> Scope7/2
  PS-Simulink Converter16/1 -> Scope7/3
  PS-Simulink Converter18/1 -> Scope8/1
  PS-Simulink Converter19/1 -> Scope9/2
  PS-Simulink Converter20/1 -> Scope9/1
  connections:
  NPN Bipolar Transistor/LConn1 -- Resistor/RConn1
  NPN Bipolar Transistor1/LConn1 -- Resistor1/RConn1
  NPN Bipolar Transistor/RConn2 -- Resistor4/LConn1 -- Resistor2/LConn1
  NPN Bipolar Transistor1/RConn2 -- Resistor5/LConn1 -- Resistor3/LConn1
  Resistor4/RConn1 -- Resistor6/LConn1 -- Op-Amp/LConn2 -- Resistor5/RConn1
  Electrical Reference/LConn1 -- Resistor2/RConn1
  Electrical Reference3/LConn1 -- Voltage Sensor1/RConn2 -- Pulse Voltage Source/RConn1 -- Solver Configuration/RConn1 -- Pulse Voltage Source2/RConn1 -- Resistor3/RConn1
  Op-Amp/LConn1 -- Voltage Sensor4/RConn2 -- Voltage Sensor/RConn2 -- Electrical Reference4/LConn1
  Op-Amp/RConn1 -- Voltage Sensor/LConn1 -- Resistor6/RConn1
  Pulse Voltage Source/LConn1 -- Resistor/LConn1 -- Voltage Sensor1/LConn1
  PS-Simulink Converter1/LConn1 -- Voltage Sensor1/RConn1
  Voltage Sensor/RConn1 -- PS-Simulink Converter/LConn1
  AC Voltage Source/LConn1 -- NPN Bipolar Transistor/RConn1
  AC Voltage Source/RConn1 -- Electrical Reference2/LConn1
  Electrical Reference1/LConn1 -- AC Voltage Source1/RConn1
  AC Voltage Source1/LConn1 -- NPN Bipolar Transistor1/RConn1
  Op-Amp1/LConn1 -- Pulse Voltage Source1/LConn1 -- Voltage Sensor3/LConn1
  Electrical Reference5/LConn1 -- Voltage Sensor2/RConn2 -- Op-Amp1/LConn2 -- Solver Configuration1/RConn1 -- Pulse Voltage Source1/RConn1 -- Voltage Sensor3/RConn2
  Voltage Sensor2/LConn1 -- Op-Amp1/RConn1
  Voltage Sensor2/RConn1 -- PS-Simulink Converter2/LConn1
  Voltage Sensor3/RConn1 -- PS-Simulink Converter3/LConn1
  Voltage Sensor4/LConn1 -- Pulse Voltage Source2/LConn1 -- Resistor1/LConn1
  Voltage Sensor4/RConn1 -- PS-Simulink Converter4/LConn1
  Solver Configuration2/RConn1 -- Electrical Reference9/LConn1 -- Resistor10/RConn1 -- Resistor8/LConn1 -- Pulse Voltage Source3/RConn1 -- Voltage Sensor6/RConn2
  Voltage Sensor6/LConn1 -- Pulse Voltage Source3/LConn1 -- Resistor7/LConn1
  Voltage Sensor5/RConn2 -- Op-Amp2/LConn2 -- Capacitor1/RConn1 -- Resistor14/RConn1 -- Capacitor/RConn1 -- Finite-Gain Op-Amp/LConn2 -- Electrical Reference10/LConn1
  Resistor10/LConn1 -- NPN Bipolar Transistor3/RConn2 -- Resistor12/LConn1
  Voltage Sensor5/LConn1 -- Diode/LConn1 -- Capacitor/LConn1 -- Resistor13/RConn1 -- Finite-Gain Op-Amp/RConn1
  Resistor12/RConn1 -- Finite-Gain Op-Amp/LConn1 -- Resistor13/LConn1 -- Resistor11/RConn1
  Resistor9/LConn1 -- NPN Bipolar Transistor2/RConn2 -- Resistor11/LConn1
  AC Voltage Source2/RConn1 -- Electrical Reference8/LConn1
  Electrical Reference7/LConn1 -- AC Voltage Source3/RConn1
  PS-Simulink Converter6/LConn1 -- Voltage Sensor6/RConn1
  AC Voltage Source2/LConn1 -- NPN Bipolar Transistor2/RConn1
  AC Voltage Source3/LConn1 -- NPN Bipolar Transistor3/RConn1
  NPN Bipolar Transistor3/LConn1 -- Resistor8/RConn1
  Voltage Sensor5/RConn1 -- PS-Simulink Converter5/LConn1
  NPN Bipolar Transistor2/LConn1 -- Resistor7/RConn1
  Electrical Reference6/LConn1 -- Resistor9/RConn1
  Resistor14/LConn1 -- Op-Amp2/LConn1 -- Capacitor1/LConn1 -- Diode/RConn1
  Voltage Sensor7/RConn1 -- PS-Simulink Converter7/LConn1
  Op-Amp2/RConn1 -- Voltage Sensor7/LConn1
  Voltage Sensor7/RConn2 -- Electrical Reference11/LConn1
  Voltage Sensor8/RConn2 -- Op-Amp3/LConn1 -- Electrical Reference16/LConn1
  Resistor18/RConn1 -- Electrical Reference15/LConn1 -- Voltage Sensor9/RConn2 -- Solver Configuration3/RConn1 -- Pulse Voltage Source4/RConn1 -- Pulse Voltage Source5/RConn1
  Resistor18/LConn1 -- NPN Bipolar Transistor5/RConn2 -- Resistor20/LConn1
  Voltage Sensor9/LConn1 -- Pulse Voltage Source4/LConn1 -- Resistor15/LConn1
  Resistor20/RConn1 -- Resistor19/RConn1 -- Resistor21/LConn1 -- Op-Amp3/LConn2
  Resistor17/LConn1 -- NPN Bipolar Transistor4/RConn2 -- Resistor19/LConn1
  Pulse Voltage Source5/LConn1 -- Resistor16/LConn1
  Resistor21/RConn1 -- Voltage Sensor8/LConn1 -- Op-Amp3/RConn1
  AC Voltage Source4/RConn1 -- Electrical Reference14/LConn1
  Voltage Sensor8/RConn1 -- PS-Simulink Converter8/LConn1
  NPN Bipolar Transistor5/RConn1 -- AC Voltage Source5/LConn1
  Electrical Reference13/LConn1 -- AC Voltage Source5/RConn1
  AC Voltage Source4/LConn1 -- NPN Bipolar Transistor4/RConn1
  PS-Simulink Converter9/LConn1 -- Voltage Sensor9/RConn1
  NPN Bipolar Transistor5/LConn1 -- Resistor16/RConn1
  Electrical Reference12/LConn1 -- Resistor17/RConn1
  NPN Bipolar Transistor4/LConn1 -- Resistor15/RConn1
  Resistor23/RConn1 -- Voltage Sensor12/RConn2 -- Op-Amp5/LConn2 -- Capacitor5/RConn1 -- Capacitor4/RConn1 -- Electrical Reference18/LConn1
  Diode2/RConn1 -- Resistor23/LConn1 -- Op-Amp5/LConn1 -- Capacitor5/LConn1
  Diode2/LConn1 -- Capacitor4/LConn1
  PS-Simulink Converter12/LConn1 -- Voltage Sensor12/RConn1
  Voltage Sensor12/LConn1 -- Op-Amp5/RConn1
  Resistor22/RConn1 -- NPN Bipolar Transistor6/LConn1
  NPN Bipolar Transistor6/RConn2 -- Voltage Sensor13/LConn1 -- Resistor24/LConn1
  Resistor22/LConn1 -- AC Voltage Source7/LConn1 -- Voltage Sensor14/LConn1
  Resistor24/RConn1 -- Voltage Sensor13/RConn2 -- Voltage Sensor14/RConn2 -- Voltage Sensor11/RConn2 -- AC Voltage Source6/RConn1 -- AC Voltage Source7/RConn1 -- Solver Configuration4/RConn1 -- Electrical Reference17/LConn1
  AC Voltage Source6/LConn1 -- Voltage Sensor11/LConn1 -- NPN Bipolar Transistor6/RConn1
  Voltage Sensor14/RConn1 -- PS-Simulink Converter11/LConn1
  Voltage Sensor11/RConn1 -- PS-Simulink Converter13/LConn1
  Voltage Sensor13/RConn1 -- PS-Simulink Converter14/LConn1
  AC Voltage Source8/LConn1 -- Voltage Sensor16/LConn1 -- CMOS AND/LConn1
  CMOS AND/LConn2 -- Voltage Sensor17/LConn1 -- AC Voltage Source9/LConn1
  Voltage Sensor15/LConn1 -- CMOS AND/RConn1
  AC Voltage Source9/RConn1 -- Voltage Sensor16/RConn2 -- Voltage Sensor15/RConn2 -- Voltage Sensor17/RConn2 -- Electrical Reference19/LConn1 -- Solver Configuration5/RConn1 -- AC Voltage Source8/RConn1
  Voltage Sensor17/RConn1 -- PS-Simulink Converter15/LConn1
  PS-Simulink Converter16/LConn1 -- Voltage Sensor15/RConn1
  Voltage Sensor16/RConn1 -- PS-Simulink Converter17/LConn1
  SPICE NMOS/RConn2 -- SPICE NMOS1/RConn2
  AC Current Source1/LConn1 -- SPICE NMOS/RConn1
  AC Current Source/LConn1 -- SPICE NMOS1/RConn1
  SPICE NMOS/RConn3 -- SPICE NMOS1/RConn3 -- SPICE NMOS2/RConn1
  SPICE NMOS2/RConn2 -- SPICE NMOS2/RConn3 -- Current Sensor/LConn1
  AC Current Source1/RConn1 -- Electrical Reference21/LConn1 -- AC Current Source/RConn1
  SPICE NMOS/LConn1 -- SPICE NMOS1/LConn1 -- SPICE NMOS2/LConn1 -- DC Voltage Source/LConn1
  Current Sensor/RConn2 -- Solver Configuration6/RConn1 -- DC Voltage Source/RConn1 -- Electrical Reference20/LConn1
  PS-Simulink Converter18/LConn1 -- Current Sensor/RConn1
  Resistor25/RConn1 -- Op-Amp4/LConn1
  AC Voltage Source10/LConn1 -- Voltage Sensor19/LConn1 -- Resistor25/LConn1
  AC Voltage Source10/RConn1 -- Solver Configuration7/RConn1 -- Voltage Sensor19/RConn2 -- Op-Amp4/LConn2 -- Voltage Sensor18/RConn2 -- Electrical Reference22/LConn1
  Voltage Sensor18/LConn1 -- Op-Amp4/RConn1
  Voltage Sensor18/RConn1 -- PS-Simulink Converter19/LConn1
  Voltage Sensor19/RConn1 -- PS-Simulink Converter20/LConn1
